simulink model "UnTrans_lin_model_Lq"  (R2015a)
settings: Solver=ode45  SolverMode=SingleTasking  StartTime=0.0  StopTime=20.0  FixedStep=Te  RelTol=1e-3
values from neighbouring files (symbols this model uses):
  A6 = [0 0 0 0 0 0 1 -0.473294023561 0 0.140107081629 0 0 ... (36 elements, 6x6)]    [ABC_buildin.mat]
  B6 = [0  0; 109.366397902  109.366397902; 0  0; -32.3752383836  -32.3752383836; 0  0; -0.505542240863  0.505542240863]    [ABC_buildin.mat]
  C6 = [1 0 0 0 0 0 0 1 0 0 0 0 ... (36 elements, 6x6)]    [ABC_buildin.mat]
  K = lqr(Hf_MIMO.a, Hf_MIMO.b, Q, R)    [ModelareArchNew.m]    (also in SSModel.m; lqrbun.mat = [-0.0544920986643  -0.0223334040175  -2.47238623528  -0.3309; try_0805.m; try_checkstuff_BUN.m = K/10)
settings Model: CovSFcnEnable=off  Creator=kha  LastModifiedBy=Maria
settings DataIOCC: SignalLoggingSaveFormat=ModelDataLogs
settings OptimizationCC: ExpressionDepthLimit=2147483647
settings DebuggingCC: UnderspecifiedInitializationDetection=Classic  MergeDetectMultiDrivingBlocksExec=none  SolverPrmCheckMsg=warning  FcnCallInpInsideContextMsg=EnableAllAsWarning  StateNameClashWarn=warning
settings GRTTargetCC: CombineOutputUpdateFcns=off  GRTInterface=on

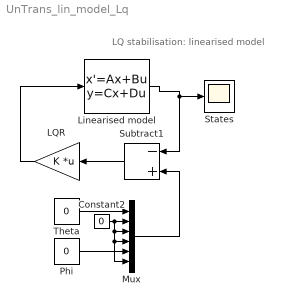
== system UnTrans_lin_model_Lq ==
  note: LQ stabilisation: linearised model
  Constant2 : Constant  Value=0
  LQR : Gain  Gain=K  Multiplication=Matrix(K*u)
  Linearised model : StateSpace  InitFcn=|  A=A6  B=B6  C=C6  D=zeros(6,2)  X0=[0 0 0.1 0 0 0]
      | UnTransPar = UnTransParams( );              
      | [A6, B6, C6] = UnTransLTIModel6(UnTransPar);
      mask Display: image( imread('Trans.jpg','jpg') )
  Mux : Mux  Inputs=6
  Phi : Constant  Value=0
  States : Scope
      settings: YMin=0  YMax=0.1  SaveName=Data_sim_l
  Subtract1 : Sum  Inputs=-+
  Theta : Constant  Value=0
  wires:
  Linearised model/1 -> Subtract1/1, States/1
  Theta/1 -> Mux/1
  Phi/1 -> Mux/5
  Constant2/1 -> Mux/6, Mux/4, Mux/3, Mux/2
  Mux/1 -> Subtract1/2
  Subtract1/1 -> LQR/1
  LQR/1 -> Linearised model/1
